simulink model "wymiennik"  (R2014a)
settings: Solver=ode45  StartTime=0.0  StopTime=9000  FixedStep=1  RelTol=1e-3
values from neighbouring files (symbols this model uses):
  godzina = str2num(text(4:5))    [komunikacja.m]
  Kp = str2num(text(17:18))+0.01*str2num(text(20:21))    [komunikacja.m]
  Ti = str2num(text(23:24))+0.01*str2num(text(26:27))    [komunikacja.m]
  To = -To    [komunikacja.m]
  Tzco = -Tzco    [komunikacja.m]
undefined symbols (not defined in the file or in its folder): c, Cw, Cwym, DiscIntNeverNeededParam, Kw, Mm
libraries: simulink x4
settings Model: Creator=asia  LastModifiedBy=lukiii
settings DataIOCC: FinalStateName=wymiennikSimState  InitialState=wymiennikSimState  SaveFinalState=on  SaveCompleteFinalSimState=on  InspectSignalLogs=on
settings DebuggingCC: UnderspecifiedInitializationDetection=Classic  StateNameClashWarn=warning

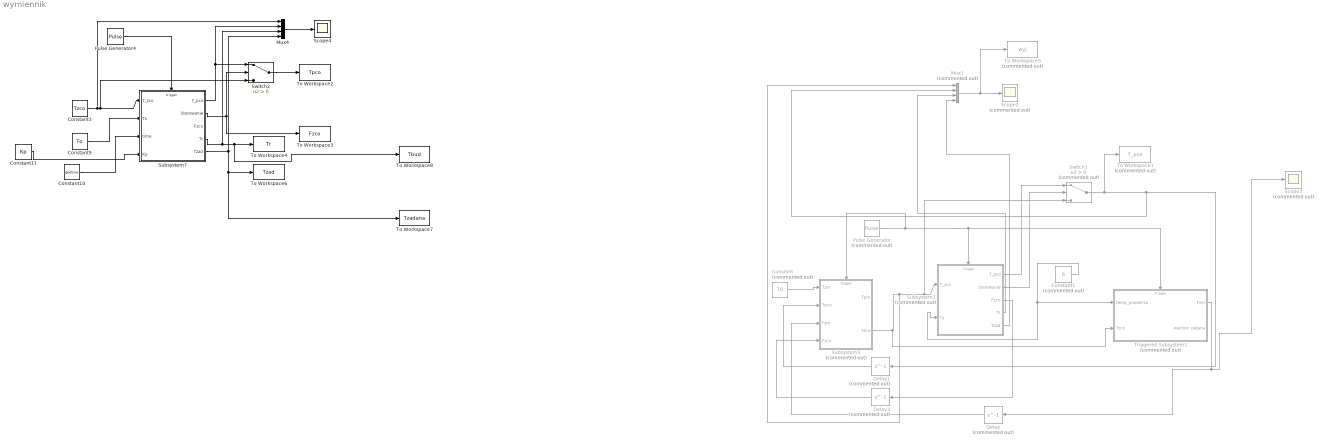
== system wymiennik ==
  Constant : Constant  Commented=on  Value=70
  Constant1 : Constant  Commented=on  Value=6
  Constant10 : Constant  Value=godzina
  Constant11 : Constant  Value=Kp
  Constant3 : Constant  Value=Tzco
  Constant9 : Constant  Value=To
  Delay : Delay  Commented=on  DelayLength=1  InitialCondition=0  SampleTime=1
  Delay1 : Delay  Commented=on  DelayLength=1  InitialCondition=0  SampleTime=1
  Delay3 : Delay  Commented=on  DelayLength=1  InitialCondition=0  SampleTime=1
  Mux1 : Mux  Commented=on
  Mux4 : Mux
  Pulse Generator : DiscretePulseGenerator  Commented=on  PulseType=Time based  Period=1  PulseWidth=50
  Pulse Generator4 : DiscretePulseGenerator  PulseType=Time based  PulseWidth=50
  Scope2 : Scope  Commented=on
      settings: TimeRange=100  YMin=0  YMax=50  SaveName=ScopeData3
  Scope3 : Scope  Commented=on
      settings: YMin=0  YMax=22.5
  Scope4 : Scope
      settings: YMin=0  YMax=40  SaveName=ScopeData4
  Subsystem1 : Subsystem  Commented=on
  Subsystem3 : Subsystem  Commented=on
  Subsystem7 : Subsystem
  Switch1 : Switch  Commented=on  Criteria=u2 > Threshold
  Switch2 : Switch  Criteria=u2 > Threshold
  To Workspace1 : ToWorkspace  Commented=on  VariableName=T_pco  SampleTime=-1
  To Workspace2 : ToWorkspace  VariableName=Tpco  SampleTime=-1
      settings: MaxDataPoints=1
  To Workspace3 : ToWorkspace  VariableName=Fzco  SampleTime=-1
      settings: MaxDataPoints=1
  To Workspace4 : ToWorkspace  VariableName=Tr  SampleTime=-1
      settings: MaxDataPoints=1
  To Workspace5 : ToWorkspace  Commented=on  VariableName=wyj  SampleTime=-1
  To Workspace6 : ToWorkspace  VariableName=Tzad  SampleTime=-1
      settings: MaxDataPoints=1
  To Workspace7 : ToWorkspace  VariableName=Tzadana  SaveFormat=Timeseries  SampleTime=-1
  To Workspace8 : ToWorkspace  VariableName=Tbud  SaveFormat=Timeseries  SampleTime=-1
  Triggered Subsystem1 : Subsystem  Commented=on  TreatAsAtomicUnit=on
  wires:
  Subsystem3/2(Tzco) -> Triggered Subsystem1/2(Tzco), Mux1/1, Switch1/3, Subsystem1/1(T_zco)
  Pulse Generator/1 -> Subsystem3/Trigger, Triggered Subsystem1/Trigger, Subsystem1/Trigger
  Constant1/1 -> Subsystem1/2(To), Triggered Subsystem1/1(temp_powietrza)
  Delay/1 -> Subsystem3/3(Fzm)
  Delay1/1 -> Subsystem3/2(Tpco)
  Mux1/1 -> To Workspace5/1, Scope2/1
  Triggered Subsystem1/1(Fzm) -> Delay/1, Scope3/1
  Constant/1 -> Subsystem3/1(Tzm)
  Switch1/1 -> To Workspace1/1, Mux1/2, Delay1/1
  Subsystem1/1(T_pco) -> Switch1/1
  Subsystem1/2(Sterowanie) -> Switch1/2
  Subsystem1/4(Tr) -> Mux1/3
  Delay3/1 -> Subsystem3/4(Fzco)
  Subsystem1/3(Fzco) -> Delay3/1
  Pulse Generator4/1 -> Subsystem7/Trigger
  Subsystem7/2(Sterowanie) -> Switch2/2, To Workspace3/1
  Subsystem7/1(T_pco) -> Mux4/2, Switch2/1
  Constant3/1 -> Mux4/1, Switch2/3, Subsystem7/1(T_zco)
  Constant9/1 -> Subsystem7/2(To)
  Switch2/1 -> To Workspace2/1
  Constant10/1 -> Subsystem7/3(time)
  Subsystem1/5(Tzad) -> Mux1/4
  Subsystem7/4(Tr) -> Mux4/3, To Workspace8/1, To Workspace4/1
  Subsystem7/5(Tzad) -> To Workspace7/1, To Workspace6/1, Mux4/4
  Constant11/1 -> Subsystem7/4(Kp)
  Mux4/1 -> Scope4/1

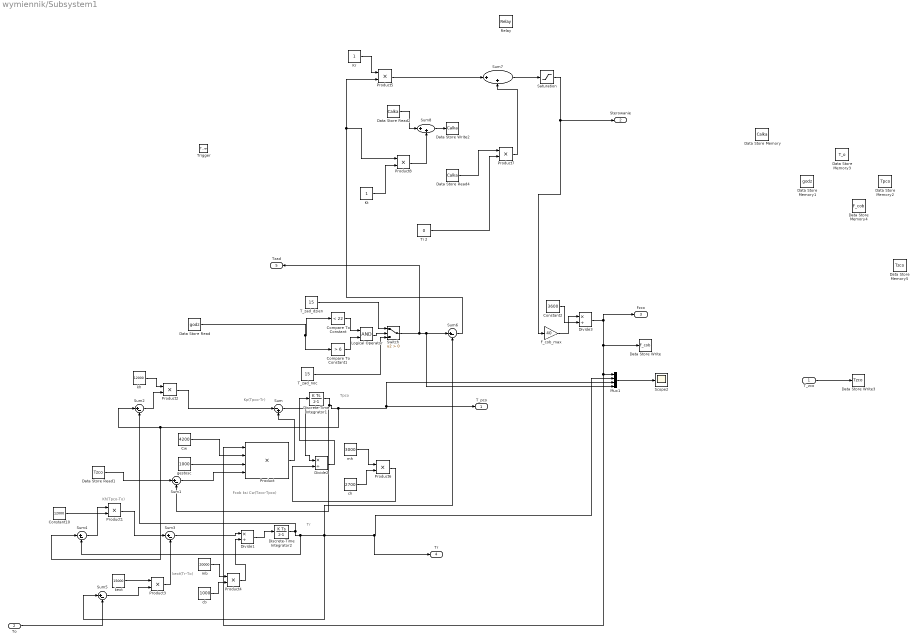
== system wymiennik/Subsystem1 ==
  note: Fcob ksi Cw(Tzco-Tpco)
  note: Kp(Tpco-Tr)
  note: Kh(Tpco-To)
  note: kext(Tr-To)
  note: Tpco
  note: Tr
  T_zco : Inport
  To : Inport  Port=2
  Trigger : TriggerPort  PortDimensions=1
  Compare To Constant : simulink/Logic and Bit Operations/Compare To Constant  relop=<  const=22  OutDataTypeStr=uint8  ZeroCross=off
  Compare To Constant1 : simulink/Logic and Bit Operations/Compare To Constant  relop=>  const=6  OutDataTypeStr=uint8  ZeroCross=off
  Constant10 : Constant  Value=12000
  Constant2 : Constant  Value=3600
  Cw : Constant  Value=4200
  Data Store Memory : DataStoreMemory  DataStoreName=Calka  ReadBeforeWriteMsg=warning  WriteAfterWriteMsg=warning  WriteAfterReadMsg=warning
  Data Store Memory1 : DataStoreMemory  DataStoreName=godz  ReadBeforeWriteMsg=warning  WriteAfterWriteMsg=warning  WriteAfterReadMsg=warning  InitialValue=10
  Data Store Memory2 : DataStoreMemory  DataStoreName=Tpco  ReadBeforeWriteMsg=warning  WriteAfterWriteMsg=warning  WriteAfterReadMsg=warning  InitialValue=10
  Data Store Memory3 : DataStoreMemory  DataStoreName=T_o  ReadBeforeWriteMsg=warning  WriteAfterWriteMsg=warning  WriteAfterReadMsg=warning
  Data Store Memory4 : DataStoreMemory  DataStoreName=F_cob  ReadBeforeWriteMsg=warning  WriteAfterWriteMsg=warning  WriteAfterReadMsg=warning  InitialValue=30
  Data Store Memory5 : DataStoreMemory  DataStoreName=Tzco  ReadBeforeWriteMsg=warning  WriteAfterWriteMsg=warning  WriteAfterReadMsg=warning  InitialValue=10
  Data Store Read : DataStoreRead  DataStoreName=godz
  Data Store Read1 : DataStoreRead  DataStoreName=Tzco
  Data Store Read2 : DataStoreRead  DataStoreName=Calka
  Data Store Read4 : DataStoreRead  DataStoreName=Calka
  Data Store Write : DataStoreWrite  DataStoreName=F_cob
  Data Store Write2 : DataStoreWrite  DataStoreName=Calka
  Data Store Write3 : DataStoreWrite  DataStoreName=Tzco
  Discrete-Time Integrator1 : DiscreteIntegrator  gainval=1  InitialCondition=20  SampleTime=-1  ICPrevOutput=DiscIntNeverNeededParam  ICPrevScaledInput=DiscIntNeverNeededParam
  Discrete-Time Integrator2 : DiscreteIntegrator  gainval=1  SampleTime=-1  ICPrevOutput=DiscIntNeverNeededParam  ICPrevScaledInput=DiscIntNeverNeededParam
  Divide1 : Product  Inputs=*/
  Divide2 : Product  Inputs=*/
  Divide3 : Product  Inputs=*/
  F_cob_max : Gain  Gain=40
  "Kr " : Constant
  "Kt " : Constant
  Logical Operator : Logic  AllPortsSameDT=off  OutDataTypeStr=boolean
  Mux1 : Mux
  Product : Product  Inputs=4  RndMeth=Zero
  Product{1..8} (8 alike) : Product  RndMeth=Zero
  Relay : Relay
  Saturation : Saturate  UpperLimit=1  LowerLimit=0
  Scope2 : Scope
      settings: YMin=0  YMax=35  SaveName=ScopeData2
  Sum : Sum  Inputs=|-+
  Sum{1..6} (6 alike) : Sum  Inputs=|+-
  Sum7 : Sum  Inputs=|++
  Sum8 : Sum  Inputs=|++
  Switch : Switch  Criteria=u2 > Threshold
  T_zad_dzien : Constant  Value=15
  T_zad_noc : Constant  Value=15
  Ti 2 : Constant  Value=0
  "cb " : Constant  Value=1000
  ch : Constant  Value=2700
  "gestosc " : Constant  Value=1000
  kext : Constant  Value=15000
  kh : Constant  Value=12000
  mb : Constant  Value=20000
  mh : Constant  Value=3000
  T_pco : Outport
  Sterowanie : Outport  Port=2
  Fzco : Outport  Port=3
  Tr : Outport  Port=4
  Tzad : Outport  Port=5
  wires:
  Sum2/1 -> Product2/2
  Product2/1 -> Sum/1
  Discrete-Time Integrator2/1 -> Sum6/2, Sum5/1, Tr/1, Mux1/2, Sum4/2, Sum2/2
  Sum3/1 -> Divide1/1
  Sum4/1 -> Product1/1
  Sum5/1 -> Product3/2
  Discrete-Time Integrator1/1 -> Sum4/1, Sum2/1, T_pco/1, Mux1/3, Sum1/2
  Compare To Constant/1 -> Logical Operator/1
  Compare To Constant1/1 -> Logical Operator/2
  Logical Operator/1 -> Switch/2
  T_zad_dzien/1 -> Switch/1
  T_zad_noc/1 -> Switch/3
  kext/1 -> Product3/1
  Product3/1 -> Sum3/2
  Constant10/1 -> Product1/2
  Product1/1 -> Sum3/1
  Divide1/1 -> Discrete-Time Integrator2/1
  "cb "/1 -> Product4/2
  mb/1 -> Product4/1
  Product4/1 -> Divide1/2
  kh/1 -> Product2/1
  Sum1/1 -> Product/4
  "gestosc "/1 -> Product/3
  Cw/1 -> Product/2
  ch/1 -> Product6/2
  mh/1 -> Product6/1
  Product6/1 -> Divide2/2
  Switch/1 -> Tzad/1, Mux1/4, Sum6/1
  F_cob_max/1 -> Divide3/1
  Mux1/1 -> Scope2/1
  Data Store Read/1 -> Compare To Constant1/1, Compare To Constant/1
  Data Store Read1/1 -> Sum1/1
  Product/1 -> Sum/2
  Sum/1 -> Divide2/1
  Divide2/1 -> Discrete-Time Integrator1/1
  Constant2/1 -> Divide3/2
  Divide3/1 -> Data Store Write/1, Product/1, Mux1/1, Fzco/1
  T_zco/1 -> Data Store Write3/1
  Product5/1 -> Sum7/1
  Sum8/1 -> Data Store Write2/1
  Sum7/1 -> Saturation/1
  "Kr "/1 -> Product5/1
  Data Store Read4/1 -> Product7/1
  Ti 2/1 -> Product7/2
  Product7/1 -> Sum7/2
  Saturation/1 -> F_cob_max/1, Sterowanie/1
  Sum6/1 -> Product5/2, Product8/1
  Product8/1 -> Sum8/2
  "Kt "/1 -> Product8/2
  Data Store Read2/1 -> Sum8/1
  To/1 -> Sum5/2

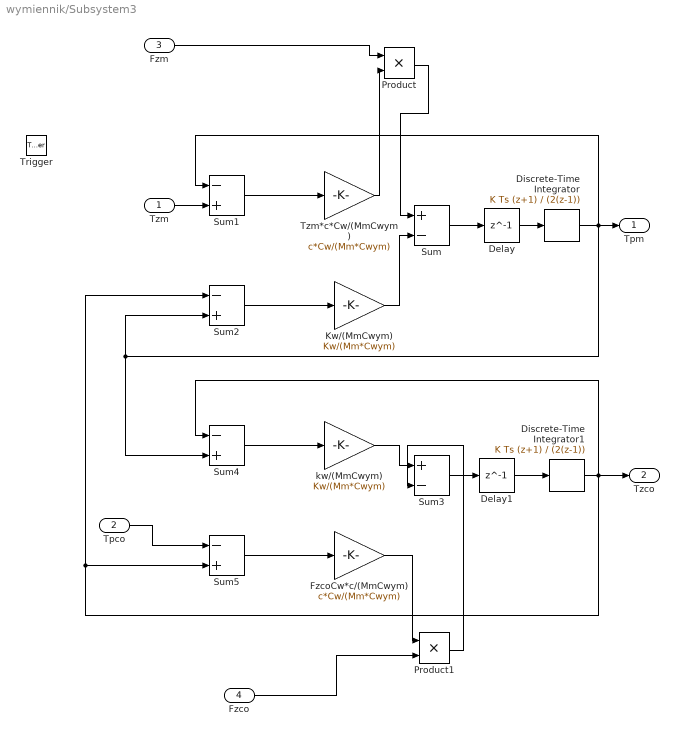
== system wymiennik/Subsystem3 ==
  Tzm : Inport
  Tpco : Inport  Port=2
  Fzm : Inport  Port=3
  Fzco : Inport  Port=4
  Trigger : TriggerPort  PortDimensions=1
  Delay : Delay  DelayLength=1  InitialCondition=0
  Delay1 : Delay  DelayLength=1  InitialCondition=0
  Discrete-Time Integrator : DiscreteIntegrator  IntegratorMethod=Integration: Trapezoidal  InitialCondition=40  SampleTime=-1  ICPrevOutput=DiscIntNeverNeededParam  ICPrevScaledInput=DiscIntNeverNeededParam
  Discrete-Time Integrator1 : DiscreteIntegrator  IntegratorMethod=Integration: Trapezoidal  InitialCondition=80  SampleTime=-1  ICPrevOutput=DiscIntNeverNeededParam  ICPrevScaledInput=DiscIntNeverNeededParam
  FzcoCw*c/(MmCwym) : Gain  Gain=c*Cw/(Mm*Cwym)
  Kw/(MmCwym) : Gain  Gain=Kw/(Mm*Cwym)
  Product : Product
  Product1 : Product  RndMeth=Zero
  Sum : Sum  Inputs=+-
  Sum{1..2,4..5} (4 alike) : Sum  Inputs=-+
  Sum3 : Sum  Inputs=+-
  Tzm*c*Cw/(MmCwym) : Gain  Gain=c*Cw/(Mm*Cwym)
  kw/(MmCwym) : Gain  Gain=Kw/(Mm*Cwym)
  Tpm : Outport
  Tzco : Outport  Port=2
  wires:
  Sum/1 -> Delay/1
  Sum2/1 -> Kw/(MmCwym)/1
  Sum1/1 -> Tzm*c*Cw/(MmCwym)/1
  Kw/(MmCwym)/1 -> Sum/2
  Tzm/1 -> Sum1/2
  Sum3/1 -> Delay1/1
  Sum5/1 -> FzcoCw*c/(MmCwym)/1
  Sum4/1 -> kw/(MmCwym)/1
  kw/(MmCwym)/1 -> Sum3/1
  Discrete-Time Integrator1/1 -> Tzco/1, Sum2/1, Sum5/2, Sum4/1
  Tpco/1 -> Sum5/1
  Discrete-Time Integrator/1 -> Sum4/2, Sum2/2, Tpm/1, Sum1/1
  Delay/1 -> Discrete-Time Integrator/1
  Delay1/1 -> Discrete-Time Integrator1/1
  Tzm*c*Cw/(MmCwym)/1 -> Product/2
  Product/1 -> Sum/1
  Fzm/1 -> Product/1
  FzcoCw*c/(MmCwym)/1 -> Product1/1
  Fzco/1 -> Product1/2
  Product1/1 -> Sum3/2

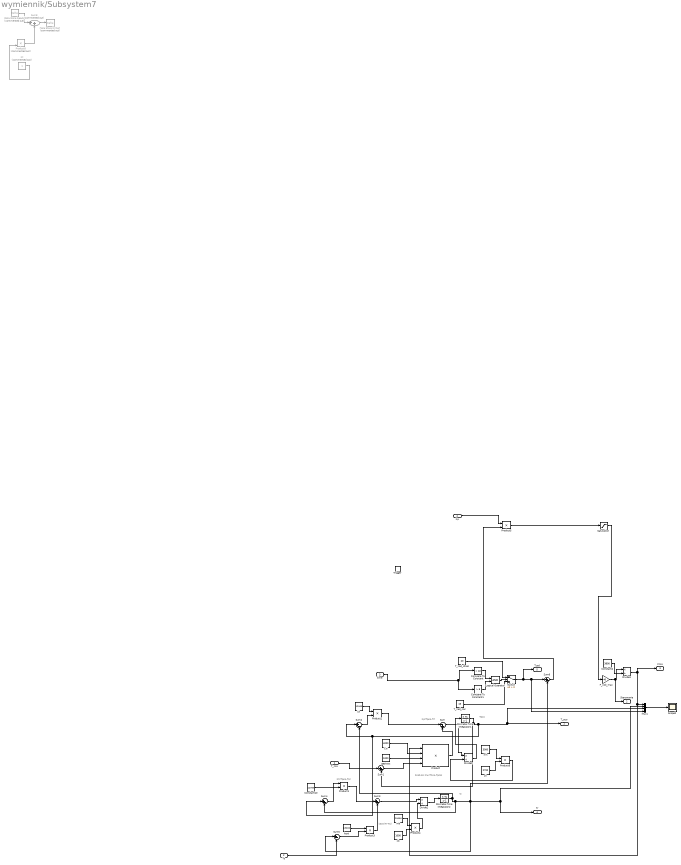
== system wymiennik/Subsystem7 ==
  note: Fcob ksi Cw(Tzco-Tpco)
  note: Kp(Tpco-Tr)
  note: Kh(Tpco-To)
  note: kext(Tr-To)
  note: Tpco
  note: Tr
  T_zco : Inport
  To : Inport  Port=2
  time : Inport  Port=3
  Kp : Inport  Port=4
  Trigger : TriggerPort  PortDimensions=1
  Compare To Constant : simulink/Logic and Bit Operations/Compare To Constant  relop=<  const=22  OutDataTypeStr=uint8  ZeroCross=off
  Compare To Constant1 : simulink/Logic and Bit Operations/Compare To Constant  relop=>  const=6  OutDataTypeStr=uint8  ZeroCross=off
  Constant10 : Constant  Value=12000
  Constant2 : Constant  Value=3600
  Cw : Constant  Value=4200
  Data Store Read2 : DataStoreRead  Commented=on  DataStoreName=Calka
  Data Store Write2 : DataStoreWrite  Commented=on  DataStoreName=Calka
  Discrete-Time Integrator1 : DiscreteIntegrator  gainval=1  InitialCondition=20  SampleTime=-1  ICPrevOutput=DiscIntNeverNeededParam  ICPrevScaledInput=DiscIntNeverNeededParam
  Discrete-Time Integrator2 : DiscreteIntegrator  gainval=1  InitialCondition=15  SampleTime=-1  ICPrevOutput=DiscIntNeverNeededParam  ICPrevScaledInput=DiscIntNeverNeededParam
  Divide1 : Product  Inputs=*/
  Divide2 : Product  Inputs=*/
  Divide3 : Product  Inputs=*/
  F_cob_max : Gain  Gain=40
  "Kt " : Constant  Commented=on
  Logical Operator : Logic  AllPortsSameDT=off  OutDataTypeStr=boolean
  Mux1 : Mux
  Product : Product  Inputs=4  RndMeth=Zero
  Product{1..6} (6 alike) : Product  RndMeth=Zero
  Product8 : Product  Commented=on  RndMeth=Zero
  Saturation : Saturate  UpperLimit=1  LowerLimit=0
  Scope2 : Scope
      settings: YMin=0  YMax=40  SaveName=ScopeData2
  Sum : Sum  Inputs=|-+
  Sum{1..6} (6 alike) : Sum  Inputs=|+-
  Sum8 : Sum  Commented=on  Inputs=|++
  Switch : Switch  Criteria=u2 > Threshold
  T_zad_dzien : Constant  Value=20
  T_zad_noc : Constant  Value=15
  "cb " : Constant  Value=1000
  ch : Constant  Value=2700
  "gestosc " : Constant  Value=1000
  kext : Constant  Value=15000
  kh : Constant  Value=12000
  mb : Constant  Value=20000
  mh : Constant  Value=3000
  T_pco : Outport
  Sterowanie : Outport  Port=2
  Fzco : Outport  Port=3
  Tr : Outport  Port=4
  Tzad : Outport  Port=5
  wires:
  Sum2/1 -> Product2/2
  Product2/1 -> Sum/1
  Discrete-Time Integrator2/1 -> Sum6/2, Sum5/1, Tr/1, Mux1/2, Sum4/2, Sum2/2
  Sum3/1 -> Divide1/1
  Sum4/1 -> Product1/1
  Sum5/1 -> Product3/2
  Discrete-Time Integrator1/1 -> Sum4/1, Sum2/1, T_pco/1, Mux1/3, Sum1/2
  Compare To Constant/1 -> Logical Operator/1
  Compare To Constant1/1 -> Logical Operator/2
  Logical Operator/1 -> Switch/2
  T_zad_dzien/1 -> Switch/1
  T_zad_noc/1 -> Switch/3
  kext/1 -> Product3/1
  Product3/1 -> Sum3/2
  Constant10/1 -> Product1/2
  Product1/1 -> Sum3/1
  Divide1/1 -> Discrete-Time Integrator2/1
  "cb "/1 -> Product4/2
  mb/1 -> Product4/1
  Product4/1 -> Divide1/2
  kh/1 -> Product2/1
  Sum1/1 -> Product/4
  "gestosc "/1 -> Product/3
  Cw/1 -> Product/2
  ch/1 -> Product6/2
  mh/1 -> Product6/1
  Product6/1 -> Divide2/2
  Switch/1 -> Tzad/1, Mux1/4, Sum6/1
  F_cob_max/1 -> Sterowanie/1, Divide3/1
  Mux1/1 -> Scope2/1
  time/1 -> Compare To Constant1/1, Compare To Constant/1
  T_zco/1 -> Sum1/1
  Product/1 -> Sum/2
  Sum/1 -> Divide2/1
  Divide2/1 -> Discrete-Time Integrator1/1
  Constant2/1 -> Divide3/2
  Divide3/1 -> Product/1, Mux1/1, Fzco/1
  Sum8/1 -> Data Store Write2/1
  Product5/1 -> Saturation/1
  Kp/1 -> Product5/1
  Saturation/1 -> F_cob_max/1
  Sum6/1 -> Product5/2
  Product8/1 -> Sum8/2
  "Kt "/1 -> Product8/2
  Data Store Read2/1 -> Sum8/1
  To/1 -> Sum5/2

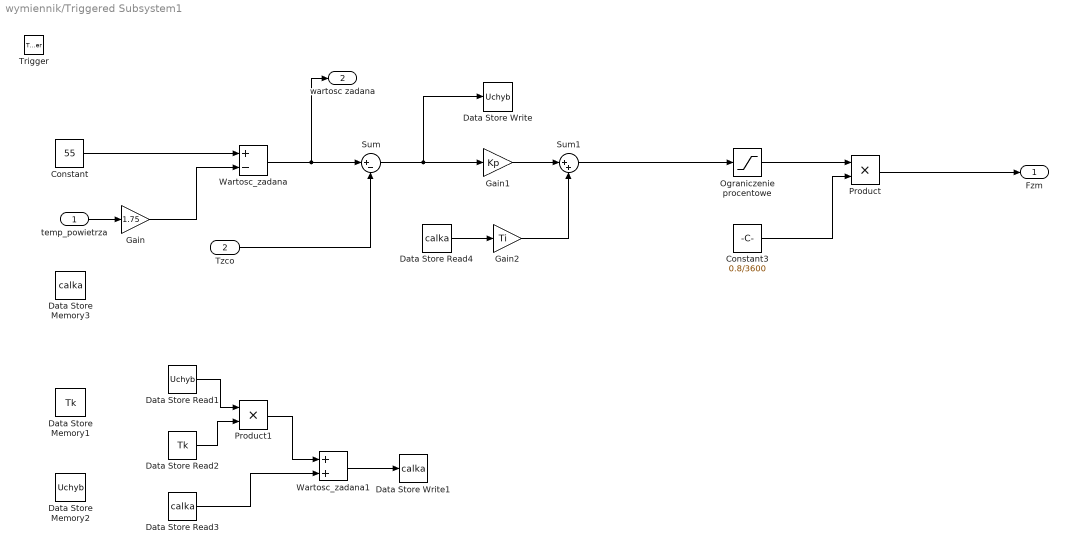
== system wymiennik/Triggered Subsystem1 ==
  temp_powietrza : Inport
  Tzco : Inport  Port=2
  Trigger : TriggerPort  PortDimensions=1
  Constant : Constant  Value=55
  Constant3 : Constant  Value=0.8/3600
  Data Store Memory1 : DataStoreMemory  DataStoreName=Tk  ReadBeforeWriteMsg=warning  WriteAfterWriteMsg=warning  WriteAfterReadMsg=warning  InitialValue=1
  Data Store Memory2 : DataStoreMemory  DataStoreName=Uchyb  ReadBeforeWriteMsg=warning  WriteAfterWriteMsg=warning  WriteAfterReadMsg=warning
  Data Store Memory3 : DataStoreMemory  DataStoreName=calka  ReadBeforeWriteMsg=warning  WriteAfterWriteMsg=warning  WriteAfterReadMsg=warning
  Data Store Read1 : DataStoreRead  DataStoreName=Uchyb
  Data Store Read2 : DataStoreRead  DataStoreName=Tk
  Data Store Read3 : DataStoreRead  DataStoreName=calka
  Data Store Read4 : DataStoreRead  DataStoreName=calka
  Data Store Write : DataStoreWrite  DataStoreName=Uchyb
  Data Store Write1 : DataStoreWrite  DataStoreName=calka
  Gain : Gain  Gain=1.75
  Gain1 : Gain  Gain=Kp
  Gain2 : Gain  Gain=Ti
  Ograniczenie procentowe : Saturate  UpperLimit=100  LowerLimit=0
  Product : Product
  Product1 : Product
  Sum : Sum  Inputs=|+-
  Sum1 : Sum  Inputs=|++
  Wartosc_zadana : Sum  Inputs=+-
  Wartosc_zadana1 : Sum
  Fzm : Outport
  wartosc zadana : Outport  Port=2
  wires:
  Data Store Read1/1 -> Product1/1
  Data Store Read3/1 -> Wartosc_zadana1/2
  Wartosc_zadana1/1 -> Data Store Write1/1
  Constant/1 -> Wartosc_zadana/1
  Gain/1 -> Wartosc_zadana/2
  Wartosc_zadana/1 -> wartosc zadana/1, Sum/1
  Sum/1 -> Data Store Write/1, Gain1/1
  Ograniczenie procentowe/1 -> Product/1
  Constant3/1 -> Product/2
  Data Store Read2/1 -> Product1/2
  Product1/1 -> Wartosc_zadana1/1
  Gain1/1 -> Sum1/1
  temp_powietrza/1 -> Gain/1
  Gain2/1 -> Sum1/2
  Data Store Read4/1 -> Gain2/1
  Product/1 -> Fzm/1
  Sum1/1 -> Ograniczenie procentowe/1
  Tzco/1 -> Sum/2
